simulink model "ModeInt"  (R2018b)
settings: Solver=FixedStepDiscrete  StartTime=0.0  StopTime=10.0  FixedStep=0.01  RelTol=1e-3
undefined symbols (not defined in the file or in its folder): c, CmprtMdHMIReqTp1, e, IfVeSMSeStNumConfig, MdReqTp1
(part 4 of 4)

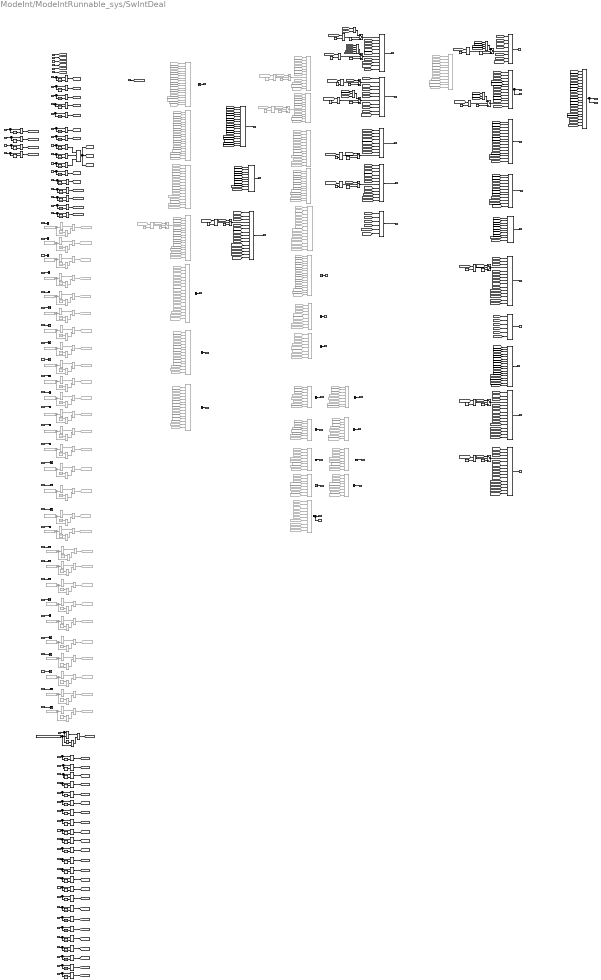
== system ModeInt/ModeIntRunnable_sys/SwIntDeal ==
  note: Note：
      | 1.修复Mode21/22/23/24自己硬线开关无法打断自己的问题。对应bug672425
  note: //local sw & memory sw & mode sw
  IsDrvStSwAct : Inport
  IsPasStSwAct : Inport  Port=2
  Is2LStSwAct : Inport  Port=3
  "Is2RStSwAct " : Inport  Port=4
  "Is3LStSwAct " : Inport  Port=5
  "Is3RStSwAct " : Inport  Port=6
  SwAcsExtLIntCnt : Inport  Port=7
  "SwAcsEntyLIntCnt " : Inport  Port=8
  "SwLfVipIntCnt " : Inport  Port=9
  SwRtVipIntCnt : Inport  Port=10
  SwLtLugIntCnt : Inport  Port=11
  SwRtLugIntCnt : Inport  Port=12
  SwAllLugIntCnt : Inport  Port=13
  SwLtRcvyIntCnt : Inport  Port=14
  SwRtRcvyIntCnt : Inport  Port=15
  AcsExtMdHMI2LRclReq : Inport  Port=16
  AcsExtMdHMI2RRclReq : Inport  Port=17
  VIPMdHMI2LRclReq : Inport  Port=18
  VIPMdHMI2RRclReq : Inport  Port=19
  RcvyMdHMI2LRclReq : Inport  Port=20
  RcvyMdHMI2RRclReq : Inport  Port=21
  LgrstOpenLtHMI2LRclReq : Inport  Port=22
  LgrstCloseLtHMI2LRclReq : Inport  Port=23
  LgrstOpenRtHMI2RRclReq : Inport  Port=24
  LgrstCloseRtHMI2RRclReq : Inport  Port=25
  passCmprtMdHMIReq : Inport  Port=26
  SRSAcsExtIntCnt : Inport  Port=27
  SRSAcsEntyIntCnt : Inport  Port=28
  SRSAllVipIntCnt : Inport  Port=29
  SRSAllLugIntCnt : Inport  Port=30
  SeStNumConfig : Inport  Port=31
  AcsEntryMdHMI2LRclReq : Inport  Port=32
  AcsEntryMdHMI2RRclReq : Inport  Port=33
  VipAllMdHMI2LRclReq : Inport  Port=34
  VipAllMdHMI2RRclReq : Inport  Port=35
  AllLugMdHMI2LRclReq : Inport  Port=36
  AllLugMdHMI2RRclReq : Inport  Port=37
  IntimacyLHMI2LRclReq : Inport  Port=38
  IntimacyRHMI2RRclReq : Inport  Port=39
  FamilyMdHMI2LRclReq : Inport  Port=40
  FamilyMdHMI2RRclReq : Inport  Port=41
  LtLugMdHMI2LRclReq : Inport  Port=42
  RtLugMdHMI2RRclReq : Inport  Port=43
  LtLyingMdHMI2LRclReq : Inport  Port=44
  RtLyingMdHMI2RRclReq : Inport  Port=45
  SRSLtFamilyIntCnt : Inport  Port=46
  SRSRtFamilyIntCnt : Inport  Port=47
  SRSIntimacyLtIntCnt : Inport  Port=48
  SRSIntimacyRtIntCnt : Inport  Port=49
  SRSLtLugIntCnt : Inport  Port=50
  SRSLtVipIntCnt : Inport  Port=51
  SRSLtLyingIntCnt : Inport  Port=52
  SRSRtLyingIntCnt : Inport  Port=53
  SRSLtRcvyIntCnt : Inport  Port=54
  SRSRtRcvyIntCnt : Inport  Port=55
  SRSRtLugIntCnt : Inport  Port=56
  SRSRtVipIntCnt : Inport  Port=57
  SRSLgrstOpenLtIntCnt : Inport  Port=58
  SRSLgrstCloseLtIntCnt : Inport  Port=59
  SRSLgrstOpenRtIntCnt : Inport  Port=60
  SRSLgrstCloseRtIntCnt : Inport  Port=61
  SwAcsExtRIntCnt : Inport  Port=62
  SwAcsEntyRIntCnt : Inport  Port=63
  SwAcsEntyBIntCnt_Val_read : Inport  Port=64
  SwAcsEntry4s2LIntCnt : Inport  Port=65
  SwAcsExit4s2LIntCnt : Inport  Port=66
  SwAcsEntry4s2RIntCnt : Inport  Port=67
  SwAcsExit4s2RIntCnt : Inport  Port=68
  AcsEntry4s2LHMI2LRclReq : Inport  Port=69
  AcsExit4s2LHMI2LRclReq : Inport  Port=70
  AcsEntry4s2RHMI2RRclReq : Inport  Port=71
  AcsExit4s2RHMI2RRclReq : Inport  Port=72
  SRSAcsEntry4s2LIntCnt : Inport  Port=73
  SRSAcsExit4s2LIntCnt : Inport  Port=74
  SRSAcsEntry4s2RIntCnt : Inport  Port=75
  SRSAcsExit4s2RIntCnt : Inport  Port=76
  SwPasReclinerEntryIntCnt : Inport  Port=77
  SwPasReclinerExitIntCnt : Inport  Port=78
  SwUnfold3LIntCnt : Inport  Port=79
  SwUnfold3RIntCnt : Inport  Port=80
  AND{,1,3..28} (28 alike) : Logic  Commented=on  AllPortsSameDT=off  OutDataTypeStr=boolean
  AND2 : Logic  AllPortsSameDT=off  OutDataTypeStr=boolean
  Constant{1,3..9,12..13,16..29,32..35} (28 alike) : Constant  Commented=on  Value=MdReqTp1.MdReqTp_Stop
  Constant10 : Constant  Commented=on  Value=IfVeSMSeStNumConfig.SeatNum7Config  OutDataTypeStr=Enum: IfVeSMSeStNumConfig
  Constant11 : Constant  Commented=on  Value=0  OutDataTypeStr=uint8
  Constant14 : Constant  Commented=on  Value=IfVeSMSeStNumConfig.SeatNum7Config  OutDataTypeStr=Enum: IfVeSMSeStNumConfig
  Constant15 : Constant  Commented=on  Value=0  OutDataTypeStr=uint8
  Constant2 : Constant  Value=CmprtMdHMIReqTp1.CmprtMdHMIReqTp_Stop  OutDataTypeStr=Enum:CmprtMdHMIReqTp1
  Constant30 : Constant  Commented=on  Value=IfVeSMSeStNumConfig.SeatNum7Config  OutDataTypeStr=Enum: IfVeSMSeStNumConfig
  Constant31 : Constant  Commented=on  Value=0  OutDataTypeStr=uint8
  Constant{36,38,40,42,44,46,48,50,52,54,56,58} (12 alike) : Constant  Value=IfVeSMSeStNumConfig.SeatNum7Config  OutDataTypeStr=Enum: IfVeSMSeStNumConfig
  Constant{37,39,41,43,45,47,49,51,53,55,57,59} (12 alike) : Constant  Value=0  OutDataTypeStr=uint8
  Equal{,1..8,14..18,27,32,59..69,79..88,97..104} (45 alike) : RelationalOperator  Operator=~=  OutDataTypeStr=boolean  RndMeth=Simplest
  Equal{10..11,19..20,23..24,28,33,35,37,39,41,43,45,47,49,51,53,55,57,71,73,75,77,90,92,94,96} (28 alike) : RelationalOperator  Commented=on  Operator=~=  OutDataTypeStr=boolean  RndMeth=Simplest
  Equal{13,105..116} (13 alike) : RelationalOperator  Operator===  OutDataTypeStr=boolean  RndMeth=Simplest
  Equal{9,12,21..22,25..26,29..31,34,36,38,40,42,44,46,48,50,52,54,56,58,70,72,74,76,78,89,91,93,95} (31 alike) : RelationalOperator  Commented=on  Operator===  OutDataTypeStr=boolean  RndMeth=Simplest
  From : From  Commented=on  GotoTag=IsDrvStSwAct
  From1 : From  Commented=on  GotoTag=IsPasStSwAct
  From{10,40,49,51,64,67,74,78,101,180,219,229,233,243} (14 alike) : From  Commented=on  GotoTag=SwAcsEntyRInt
  From{6,20,30,32,35,63,76,100,134,158,173,183,211..212} (14 alike) : From  Commented=on  GotoTag=SwAcsEntyLInt
  From102 : From  Commented=on  GotoTag=SRSAcsExtInt
  From103 : From  Commented=on  GotoTag=SRSAcsEntyInt
  From104 : From  Commented=on  GotoTag=SRSAllVipInt
  From105 : From  Commented=on  GotoTag=SRSAllLugInt
  From106 : From  Commented=on  GotoTag=AcsExtMdHMI2LStop
  From107 : From  Commented=on  GotoTag=VIPMdHMI2LStop
  From108 : From  Commented=on  GotoTag=RcvyMdHMI2LStop
  From109 : From  Commented=on  GotoTag=AcsExtMdHMI2RStop
  From{11,34,53,55,73,79,99,115,181,201,204,227,230,247} (14 alike) : From  Commented=on  GotoTag=SwAcsExtRInt
  From110 : From  Commented=on  GotoTag=VIPMdHMI2RStop
  From111 : From  Commented=on  GotoTag=RcvyMdHMI2RStop
  From{54,69,71,81,112..114,116,133,192,198,220,231,234} (14 alike) : From  Commented=on  GotoTag=SwAcsEntyBInt
  From117 : From  Commented=on  GotoTag=AcsEntryMdHMI2LStop
  From118 : From  Commented=on  GotoTag=AcsEntryMdHMI2RStop
  From119 : From  Commented=on  GotoTag=VipAllMdHMI2LStop
  From{12,23,36,61,137,164,178,186,195..196,207,238,271,279} (14 alike) : From  Commented=on  GotoTag=SwLtRcvyInt
  From120 : From  Commented=on  GotoTag=VipAllMdHMI2RStop
  From121 : From  Commented=on  GotoTag=AllLugMdHMI2LStop
  From122 : From  Commented=on  GotoTag=AllLugMdHMI2RStop
  From123 : From  Commented=on  GotoTag=IntimacyLHMI2LStop
  From{2,16,28,57,124,153,155,159,166,169,191,237,267,277} (14 alike) : From  Commented=on  GotoTag=Is2LStSwAct
  From125 : From  Commented=on  GotoTag=FamilyMdHMI2LStop
  From126 : From  Commented=on  GotoTag=FamilyMdHMI2RStop
  From127 : From  Commented=on  GotoTag=LtLugMdHMI2LStop
  From128 : From  Commented=on  GotoTag=RtLugMdHMI2RStop
  From129 : From  Commented=on  GotoTag=LtLyingMdHMI2LStop
  From{13,24,46,66,138,165,179,187,203,214,222,286,294..295} (14 alike) : From  Commented=on  GotoTag=SwRtRcvyInt
  From130 : From  Commented=on  GotoTag=RtLyingMdHMI2RStop
  From{5,26,52,131,156} (5 alike) : From  Commented=on  GotoTag=Is3RStSwAct
  From{3,17,38,62,132,152,154,167,170,199,218,270,284,292} (14 alike) : From  Commented=on  GotoTag=Is2RStSwAct
  From{7,21,31,39,44,60,135,160,163,174,184,190,194,206,236,266,278} (17 alike) : From  Commented=on  GotoTag=SwLfVipInt
  From{8,22,42,58..59,65,91,136,161,175,185,202,213,221,272,285,293} (17 alike) : From  Commented=on  GotoTag=SwRtVipInt
  From139 : From  Commented=on  GotoTag=SRSLtFamilyInt
  From14 : From  Commented=on  GotoTag=IsDrvStSwAct
  From140 : From  Commented=on  GotoTag=SRSRtFamilyInt
  From141 : From  Commented=on  GotoTag=SRSIntimacyLtInt
  From142 : From  Commented=on  GotoTag=SRSLtLugInt
  From{77,82,84,86,88,90,93..94,96,98,143,151,168,182,188,197,205,210,217,225,269,275,283,291} (24 alike) : From  Commented=on  GotoTag=passCmprtMdHMIStop
  From144 : From  Commented=on  GotoTag=SRSLtLyingInt
  From145 : From  Commented=on  GotoTag=SRSRtLyingInt
  From146 : From  Commented=on  GotoTag=SRSLtRcvyInt
  From147 : From  Commented=on  GotoTag=SRSRtRcvyInt
  From148 : From  Commented=on  GotoTag=SRSRtLugInt
  From149 : From  Commented=on  GotoTag=SRSLgrstOpenLtInt
  From15 : From  Commented=on  GotoTag=IsPasStSwAct
  From150 : From  Commented=on  GotoTag=LgrstOpenLtHMI2LStop
  From{18..19,29,45,48,68,75,92,157,172,177,193,200,226} (14 alike) : From  Commented=on  GotoTag=SwAcsExtLInt
  From162 : From  Commented=on  GotoTag=SeStNumConfig
  From{4,25,37,47,97,171} (6 alike) : From  Commented=on  GotoTag=Is3LStSwAct
  From{9,33,43,50,70,176,189,228,232,235} (10 alike) : From  Commented=on  GotoTag=SwLtLugInt
  From208 : From  Commented=on  GotoTag=SRSLgrstCloseLtInt
  From209 : From  Commented=on  GotoTag=LgrstCloseLtHMI2LStop
  From215 : From  Commented=on  GotoTag=SRSLgrstOpenRtInt
  From216 : From  Commented=on  GotoTag=LgrstOpenRtHMI2RStop
  From223 : From  Commented=on  GotoTag=SRSLgrstCloseRtInt
  From224 : From  Commented=on  GotoTag=LgrstCloseRtHMI2RStop
  From239 : From  Commented=on  GotoTag=AcsEntry4s2LHMI2LStop
  From{240,245,250,254,258,260,280,297,301} (9 alike) : From  Commented=on  GotoTag=SwAcsEntry4s2LInt
  From{241,246,251,255,259,261,276,296,300} (9 alike) : From  Commented=on  GotoTag=SwAcsExit4s2LInt
  From{242,248,252,256,262,264,287,299,302} (9 alike) : From  Commented=on  GotoTag=SwAcsEntry4s2RInt
  From{244,249,253,257,263,265,288,298,303} (9 alike) : From  Commented=on  GotoTag=SwAcsExit4s2RInt
  From268 : From  Commented=on  GotoTag=AcsExit4s2RHMI2RStop
  From27 : From  Commented=on  GotoTag=IntimacyRHMI2RStop
  From273 : From  Commented=on  GotoTag=SRSAcsExit4s2RInt
  From274 : From  Commented=on  GotoTag=SRSAcsEntry4s2LInt
  From281 : From  Commented=on  GotoTag=SRSAcsExit4s2LInt
  From282 : From  Commented=on  GotoTag=AcsExit4s2LHMI2LStop
  From289 : From  Commented=on  GotoTag=AcsEntry4s2RHMI2RStop
  From290 : From  Commented=on  GotoTag=SRSAcsEntry4s2RInt
  From41 : From  Commented=on  GotoTag=IsDrvStSwAct
  From56 : From  Commented=on  GotoTag=SwRtLugInt
  From72 : From  Commented=on  GotoTag=SwAllLugInt
  From80 : From  Commented=on  GotoTag=IsPasStSwAct
  From83 : From  Commented=on  GotoTag=SRSRtVipInt
  From85 : From  Commented=on  GotoTag=SRSLtVipInt
  From87 : From  Commented=on  GotoTag=SeStNumConfig
  From89 : From  Commented=on  GotoTag=SeStNumConfig
  From95 : From  Commented=on  GotoTag=SRSIntimacyRtInt
  Goto15 : Goto  Commented=on  GotoTag=AcsExtMdHMI2LStop
  Goto16 : Goto  Commented=on  GotoTag=AcsExtMdHMI2RStop
  Goto22 : Goto  Commented=on  GotoTag=VIPMdHMI2LStop
  Goto23 : Goto  Commented=on  GotoTag=VIPMdHMI2RStop
  Goto24 : Goto  Commented=on  GotoTag=RcvyMdHMI2LStop
  Goto25 : Goto  Commented=on  GotoTag=RcvyMdHMI2RStop
  Goto26 : Goto  Commented=on  GotoTag=LgrstOpenLtHMI2LStop
  Goto27 : Goto  Commented=on  GotoTag=LgrstCloseLtHMI2LStop
  Goto29 : Goto  Commented=on  GotoTag=AcsEntryMdHMI2LStop
  Goto30 : Goto  Commented=on  GotoTag=AcsEntryMdHMI2RStop
  Goto31 : Goto  Commented=on  GotoTag=VipAllMdHMI2LStop
  Goto32 : Goto  Commented=on  GotoTag=VipAllMdHMI2RStop
  Goto33 : Goto  Commented=on  GotoTag=AllLugMdHMI2LStop
  Goto34 : Goto  Commented=on  GotoTag=AllLugMdHMI2RStop
  Goto35 : Goto  Commented=on  GotoTag=IntimacyLHMI2LStop
  Goto36 : Goto  Commented=on  GotoTag=IntimacyRHMI2RStop
  Goto37 : Goto  Commented=on  GotoTag=FamilyMdHMI2LStop
  Goto38 : Goto  Commented=on  GotoTag=FamilyMdHMI2RStop
  Goto39 : Goto  Commented=on  GotoTag=LtLugMdHMI2LStop
  Goto40 : Goto  Commented=on  GotoTag=RtLugMdHMI2RStop
  Goto41 : Goto  Commented=on  GotoTag=LtLyingMdHMI2LStop
  Goto42 : Goto  Commented=on  GotoTag=RtLyingMdHMI2RStop
  Goto54 : Goto  Commented=on  GotoTag=LgrstOpenRtHMI2RStop
  Goto55 : Goto  Commented=on  GotoTag=LgrstCloseRtHMI2RStop
  Goto68 : Goto  Commented=on  GotoTag=AcsEntry4s2LHMI2LStop
  Goto69 : Goto  Commented=on  GotoTag=AcsExit4s2LHMI2LStop
  Goto70 : Goto  Commented=on  GotoTag=AcsEntry4s2RHMI2RStop
  Goto71 : Goto  Commented=on  GotoTag=AcsExit4s2RHMI2RStop
  Ground{,1..15} (16 alike) : Ground
  OR : Logic  Commented=on  Operator=OR  Inputs=20  AllPortsSameDT=off  OutDataTypeStr=boolean
  OR1 : Logic  Commented=on  Operator=OR  Inputs=18  AllPortsSameDT=off  OutDataTypeStr=boolean
  OR10 : Logic  Commented=on  Operator=OR  Inputs=15  AllPortsSameDT=off  OutDataTypeStr=boolean
  OR{11,16..24} (10 alike) : Logic  Commented=on  Operator=OR  Inputs=8  AllPortsSameDT=off  OutDataTypeStr=boolean
  OR12 : Logic  Operator=OR  Inputs=3  AllPortsSameDT=off  OutDataTypeStr=boolean
  OR13 : Logic  Commented=on  Operator=OR  Inputs=17  AllPortsSameDT=off  OutDataTypeStr=boolean
  OR14 : Logic  Commented=on  Operator=OR  Inputs=17  AllPortsSameDT=off  OutDataTypeStr=boolean
  OR15 : Logic  Commented=on  Operator=OR  Inputs=15  AllPortsSameDT=off  OutDataTypeStr=boolean
  OR2 : Logic  Commented=on  Operator=OR  Inputs=16  AllPortsSameDT=off  OutDataTypeStr=boolean
  OR25 : Logic  Commented=on  Operator=OR  Inputs=10  AllPortsSameDT=off  OutDataTypeStr=boolean
  OR26 : Logic  Operator=OR  Inputs=17  AllPortsSameDT=off  OutDataTypeStr=boolean
  OR27 : Logic  Operator=OR  Inputs=10  AllPortsSameDT=off  OutDataTypeStr=boolean
  OR{28,40,43,45..46} (5 alike) : Logic  Operator=OR  Inputs=15  AllPortsSameDT=off  OutDataTypeStr=boolean
  OR29 : Logic  Operator=OR  AllPortsSameDT=off  OutDataTypeStr=boolean
  OR3 : Logic  Commented=on  Operator=OR  Inputs=17  AllPortsSameDT=off  OutDataTypeStr=boolean
  OR30 : Logic  Operator=OR  Inputs=5  AllPortsSameDT=off  OutDataTypeStr=boolean
  OR31 : Logic  Operator=OR  Inputs=11  AllPortsSameDT=off  OutDataTypeStr=boolean
  OR32 : Logic  Operator=OR  Inputs=17  AllPortsSameDT=off  OutDataTypeStr=boolean
  OR33 : Logic  Operator=OR  Inputs=11  AllPortsSameDT=off  OutDataTypeStr=boolean
  OR34 : Logic  Operator=OR  Inputs=9  AllPortsSameDT=off  OutDataTypeStr=boolean
  OR35 : Logic  Operator=OR  Inputs=12  AllPortsSameDT=off  OutDataTypeStr=boolean
  OR36 : Logic  Operator=OR  Inputs=6  AllPortsSameDT=off  OutDataTypeStr=boolean
  OR37 : Logic  Operator=OR  Inputs=8  AllPortsSameDT=off  OutDataTypeStr=boolean
  OR38 : Logic  Operator=OR  Inputs=4  AllPortsSameDT=off  OutDataTypeStr=boolean
  OR39 : Logic  Operator=OR  Inputs=13  AllPortsSameDT=off  OutDataTypeStr=boolean
  OR4 : Logic  Commented=on  Operator=OR  Inputs=12  AllPortsSameDT=off  OutDataTypeStr=boolean
  OR41 : Logic  Operator=OR  Inputs=12  AllPortsSameDT=off  OutDataTypeStr=boolean
  OR42 : Logic  Operator=OR  Inputs=10  AllPortsSameDT=off  OutDataTypeStr=boolean
  OR44 : Logic  Operator=OR  Inputs=6  AllPortsSameDT=off  OutDataTypeStr=boolean
  OR47 : Logic  Operator=OR  Inputs=3  AllPortsSameDT=off  OutDataTypeStr=boolean
  OR48 : Logic  Operator=OR  Inputs=3  AllPortsSameDT=off  OutDataTypeStr=boolean
  OR49 : Logic  Operator=OR  Inputs=20  AllPortsSameDT=off  OutDataTypeStr=boolean
  OR5 : Logic  Commented=on  Operator=OR  Inputs=12  AllPortsSameDT=off  OutDataTypeStr=boolean
  OR6 : Logic  Commented=on  Operator=OR  Inputs=13  AllPortsSameDT=off  OutDataTypeStr=boolean
  OR7 : Logic  Commented=on  Operator=OR  Inputs=13  AllPortsSameDT=off  OutDataTypeStr=boolean
  OR8 : Logic  Commented=on  Operator=OR  Inputs=14  AllPortsSameDT=off  OutDataTypeStr=boolean
  OR9 : Logic  Commented=on  Operator=OR  Inputs=12  AllPortsSameDT=off  OutDataTypeStr=boolean
  Switch : Switch  Commented=on  Criteria=u2 > Threshold
  Switch1 : Switch  Commented=on  Criteria=u2 > Threshold
  Switch{3..13,15} (12 alike) : Switch  Criteria=u2 > Threshold
  Switch2 : Switch  Commented=on  Criteria=u2 > Threshold
  Terminator{,1..27} (28 alike) : Terminator
  Unit Delay{,1..8,12..15,34..44,49..60,65..72} (44 alike) : UnitDelay  SampleTime=-1
  Unit Delay{9..10,16..33,45..48,61..64} (28 alike) : UnitDelay  Commented=on  InitialCondition=e  SampleTime=-1
  Unit Delay11 : UnitDelay  InitialCondition=c  SampleTime=-1
  SwIntAcsEnty : Outport
  SwIntAcsExt : Outport  Port=2
  SwIntLfVip : Outport  Port=3
  SwIntRtVip : Outport  Port=4
  SwIntLfLug : Outport  Port=5
  SwIntRtLug : Outport  Port=6
  SwIntLfRcvy : Outport  Port=7
  SwIntRtRcvy : Outport  Port=8
  SwIntAllVip : Outport  Port=9
  SwIntAllLug : Outport  Port=10
  SwIntLtFamily : Outport  Port=11
  SwIntRtFamily : Outport  Port=12
  SwIntIntimacyLt : Outport  Port=13
  SwIntLtLying : Outport  Port=14
  SwIntRtLying : Outport  Port=15
  SwIntIntimacyRt : Outport  Port=16
  SwIntLgrstOpenLt : Outport  Port=17
  SwIntLgrstCloseLt : Outport  Port=18
  SwIntLgrstOpenRt : Outport  Port=19
  SwIntLgrstCloseRt : Outport  Port=20
  SwIntAcsEntry4s2L : Outport  Port=21
  SwIntAcsExit4s2L : Outport  Port=22
  SwIntAcsEntry4s2R : Outport  Port=23
  SwIntAcsExit4s2R : Outport  Port=24
  SwIntAcsEntryAll4sBwd : Outport  Port=25
  SwIntAcsEntryAll4sFwd : Outport  Port=26
  SwIntPasReclinerEntry : Outport  Port=27
  SwIntPasReclinerExit : Outport  Port=28
  SwIntUnfold3L : Outport  Port=29
  SwIntUnfold3R : Outport  Port=30
  SwIntLfVipOut : Outport  Port=31
  SwIntRtVipOut : Outport  Port=32
  SwIntAllVipOut : Outport  Port=33
  SwIntBig4Seat : Outport  Port=34
  SwIntExVIPR : Outport  Port=35
  SwIntExVIPROut : Outport  Port=36
  SwIntWholeVehMem1 : Outport  Port=37
  SwIntWholeVehMem2 : Outport  Port=38
  wires:
  IsDrvStSwAct/1 -> [IsDrvStSwAct]
  IsPasStSwAct/1 -> [IsPasStSwAct]
  Is2LStSwAct/1 -> [Is2LStSwAct]
  "Is2RStSwAct "/1 -> [Is2RStSwAct]
  "Is3LStSwAct "/1 -> [Is3LStSwAct]
  "Is3RStSwAct "/1 -> [Is3RStSwAct]
  From/1 -> OR/1
  From1/1 -> OR/2
  From2/1 -> OR/3
  From3/1 -> OR/4
  From4/1 -> OR/5
  From5/1 -> OR/6
  From14/1 -> OR1/1
  From15/1 -> OR1/2
  From16/1 -> OR1/3
  From17/1 -> OR1/4
  From52/1 -> OR5/1
  From57/1 -> OR6/1
  From62/1 -> OR7/1
  Equal2/1 -> [SwLfVipInt]
  "SwLfVipIntCnt "/1 -> Equal2/1, Unit Delay2/1
  Unit Delay2/1 -> Equal2/2
  SwRtVipIntCnt/1 -> Unit Delay3/1, Equal3/1
  Unit Delay3/1 -> Equal3/2
  Equal3/1 -> [SwRtVipInt]
  SwLtLugIntCnt/1 -> Equal4/1, Unit Delay4/1
  Unit Delay4/1 -> Equal4/2
  SwRtLugIntCnt/1 -> Unit Delay5/1, Equal5/1
  Unit Delay5/1 -> Equal5/2
  Unit Delay6/1 -> Equal6/2
  SwAllLugIntCnt/1 -> Unit Delay6/1, Equal6/1
  Equal7/1 -> [SwLtRcvyInt]
  SwLtRcvyIntCnt/1 -> Unit Delay7/1, Equal7/1
  Unit Delay7/1 -> Equal7/2
  Equal8/1 -> [SwRtRcvyInt]
  SwRtRcvyIntCnt/1 -> Unit Delay8/1, Equal8/1
  Unit Delay8/1 -> Equal8/2
  Constant8/1 -> Equal10/2, Equal9/2
  Unit Delay9/1 -> Equal10/1
  Equal9/1 -> AND/1
  Equal10/1 -> AND/2
  AND/1 -> Goto15/1
  Constant1/1 -> Equal11/2, Equal12/2
  AND1/1 -> Goto16/1
  Unit Delay10/1 -> Equal11/1
  Equal11/1 -> AND1/2
  Equal12/1 -> AND1/1
  passCmprtMdHMIReq/1 -> Unit Delay11/1, Equal13/1
  Constant2/1 -> Equal14/2, Equal13/2
  Unit Delay11/1 -> Equal14/1
  Equal13/1 -> AND2/1
  Equal14/1 -> AND2/2
  AND2/1 -> [passCmprtMdHMIStop]
  Unit Delay15/1 -> Equal18/2
  SRSAllVipIntCnt/1 -> Unit Delay14/1, Equal17/1
  SRSAllLugIntCnt/1 -> Unit Delay15/1, Equal18/1
  SRSAcsEntyIntCnt/1 -> Unit Delay13/1, Equal16/1
  SRSAcsExtIntCnt/1 -> Unit Delay12/1, Equal15/1
  Unit Delay14/1 -> Equal17/2
  Unit Delay13/1 -> Equal16/2
  Equal18/1 -> [SRSAllLugInt]
  Equal15/1 -> [SRSAcsExtInt]
  Unit Delay12/1 -> Equal15/2
  Equal17/1 -> [SRSAllVipInt]
  Equal16/1 -> [SRSAcsEntyInt]
  Equal22/1 -> AND3/1
  AND4/1 -> Goto23/1
  AND3/1 -> Goto22/1
  Constant4/1 -> Equal19/2, Equal22/2
  Equal19/1 -> AND3/2
  Unit Delay16/1 -> Equal20/1
  Equal21/1 -> AND4/1
  Equal20/1 -> AND4/2
  Unit Delay17/1 -> Equal19/1
  Constant3/1 -> Equal20/2, Equal21/2
  Equal25/1 -> AND6/1
  Constant5/1 -> Equal24/2, Equal25/2
  Unit Delay19/1 -> Equal23/1
  Constant6/1 -> Equal23/2, Equal26/2
  AND5/1 -> Goto24/1
  Equal23/1 -> AND5/2
  Unit Delay18/1 -> Equal24/1
  Equal26/1 -> AND5/1
  AND6/1 -> Goto25/1
  Equal24/1 -> AND6/2
  AND7/1 -> Goto29/1
  Equal30/1 -> AND7/1
  Equal28/1 -> AND7/2
  Constant7/1 -> Equal28/2, Equal30/2
  Unit Delay20/1 -> Equal28/1
  Unit Delay21/1 -> Equal33/1
  Constant9/1 -> Equal33/2, Equal34/2
  Equal34/1 -> AND8/1
  Equal33/1 -> AND8/2
  AND8/1 -> Goto30/1
  AND9/1 -> Goto31/1
  Constant12/1 -> Equal35/2, Equal36/2
  Equal36/1 -> AND9/1
  Unit Delay22/1 -> Equal35/1
  Equal35/1 -> AND9/2
  Constant13/1 -> Equal37/2, Equal38/2
  AND10/1 -> Goto32/1
  Unit Delay23/1 -> Equal37/1
  Equal38/1 -> AND10/1
  Equal37/1 -> AND10/2
  AND11/1 -> Goto33/1
  Equal39/1 -> AND11/2
  Unit Delay24/1 -> Equal39/1
  Equal40/1 -> AND11/1
  Constant20/1 -> Equal39/2, Equal40/2
  Constant21/1 -> Equal41/2, Equal42/2
  Equal42/1 -> AND12/1
  Equal41/1 -> AND12/2
  Unit Delay25/1 -> Equal41/1
  AND12/1 -> Goto34/1
  Equal44/1 -> AND13/1
  Unit Delay26/1 -> Equal43/1
  Constant22/1 -> Equal43/2, Equal44/2
  AND13/1 -> Goto35/1
  Equal43/1 -> AND13/2
  Equal45/1 -> AND14/2
  Constant23/1 -> Equal45/2, Equal46/2
  Unit Delay27/1 -> Equal45/1
  AND14/1 -> Goto36/1
  Equal46/1 -> AND14/1
  Equal48/1 -> AND15/1
  AND15/1 -> Goto37/1
  Unit Delay28/1 -> Equal47/1
  Constant24/1 -> Equal47/2, Equal48/2
  Equal47/1 -> AND15/2
  Equal50/1 -> AND16/1
  AND16/1 -> Goto38/1
  Equal49/1 -> AND16/2
  Unit Delay29/1 -> Equal49/1
  Constant25/1 -> Equal49/2, Equal50/2
  Constant26/1 -> Equal51/2, Equal52/2
  Unit Delay30/1 -> Equal51/1
  AND17/1 -> Goto39/1
  Equal51/1 -> AND17/2
  Equal52/1 -> AND17/1
  AND18/1 -> Goto40/1
  Unit Delay31/1 -> Equal53/1
  Equal54/1 -> AND18/1
  Equal53/1 -> AND18/2
  Constant27/1 -> Equal53/2, Equal54/2
  Constant28/1 -> Equal55/2, Equal56/2
  Equal55/1 -> AND19/2
  Unit Delay32/1 -> Equal55/1
  Equal56/1 -> AND19/1
  AND19/1 -> Goto41/1
  Constant29/1 -> Equal57/2, Equal58/2
  Equal57/1 -> AND20/2
  Unit Delay33/1 -> Equal57/1
  Equal58/1 -> AND20/1
  AND20/1 -> Goto42/1
  Equal59/1 -> [SRSLtFamilyInt]
  SRSLtFamilyIntCnt/1 -> Unit Delay34/1, Equal59/1
  Unit Delay34/1 -> Equal59/2
  Unit Delay35/1 -> Equal60/2
  Equal60/1 -> [SRSRtFamilyInt]
  SRSRtFamilyIntCnt/1 -> Unit Delay35/1, Equal60/1
  Unit Delay36/1 -> Equal61/2
  SRSIntimacyLtIntCnt/1 -> Unit Delay36/1, Equal61/1
  Equal61/1 -> [SRSIntimacyLtInt]
  Equal62/1 -> [SRSLtLugInt]
  SRSLtLugIntCnt/1 -> Unit Delay37/1, Equal62/1
  Unit Delay37/1 -> Equal62/2
  Unit Delay38/1 -> Equal63/2
  SRSLtVipIntCnt/1 -> Unit Delay38/1, Equal63/1
  Equal63/1 -> [SRSLtVipInt]
  Equal64/1 -> [SRSLtLyingInt]
  SRSLtLyingIntCnt/1 -> Unit Delay39/1, Equal64/1
  Unit Delay39/1 -> Equal64/2
  Unit Delay40/1 -> Equal65/2
  Equal65/1 -> [SRSRtLyingInt]
  SRSRtLyingIntCnt/1 -> Unit Delay40/1, Equal65/1
  SRSLtRcvyIntCnt/1 -> Unit Delay41/1, Equal66/1
  Equal66/1 -> [SRSLtRcvyInt]
  Unit Delay41/1 -> Equal66/2
  SRSRtRcvyIntCnt/1 -> Unit Delay42/1, Equal67/1
  Unit Delay42/1 -> Equal67/2
  Equal67/1 -> [SRSRtRcvyInt]
  Unit Delay43/1 -> Equal68/2
  Equal68/1 -> [SRSRtLugInt]
  SRSRtLugIntCnt/1 -> Unit Delay43/1, Equal68/1
  Unit Delay44/1 -> Equal69/2
  Equal69/1 -> [SRSRtVipInt]
  SRSRtVipIntCnt/1 -> Unit Delay44/1, Equal69/1
  From153/1 -> OR13/1
  From154/1 -> OR13/2
  From171/1 -> OR14/3
  From170/1 -> OR14/2
  From169/1 -> OR14/1
  From159/1 -> OR15/1
  From167/1 -> OR15/2
  From191/1 -> OR16/1
  From199/1 -> OR17/1
  "SwAcsEntyLIntCnt "/1 -> Unit Delay1/1, Equal1/1
  Unit Delay1/1 -> Equal1/2
  Equal1/1 -> [SwAcsEntyLInt]
  Unit Delay/1 -> Equal/2
  SwAcsExtLIntCnt/1 -> Unit Delay/1, Equal/1
  Equal/1 -> [SwAcsExtLInt]
  From156/1 -> OR13/4
  From97/1 -> OR13/3
  From131/1 -> OR14/4
  Equal72/1 -> AND21/1
  Unit Delay45/1 -> Equal71/1
  Equal71/1 -> AND21/2
  Constant32/1 -> Equal71/2, Equal72/2
  AND21/1 -> Goto26/1
  Constant33/1 -> Equal73/2, Equal74/2
  Equal73/1 -> AND22/2
  Equal74/1 -> AND22/1
  Unit Delay46/1 -> Equal73/1
  AND22/1 -> Goto27/1
  Constant34/1 -> Equal75/2, Equal76/2
  Equal75/1 -> AND23/2
  Equal76/1 -> AND23/1
  Unit Delay47/1 -> Equal75/1
  AND23/1 -> Goto54/1
  Unit Delay48/1 -> Equal77/1
  AND24/1 -> Goto55/1
  Equal78/1 -> AND24/1
  Equal77/1 -> AND24/2
  Constant35/1 -> Equal77/2, Equal78/2
  Unit Delay49/1 -> Equal79/2
  SRSIntimacyRtIntCnt/1 -> Unit Delay49/1, Equal79/1
  Equal79/1 -> [SRSIntimacyRtInt]
  Equal80/1 -> [SRSLgrstOpenLtInt]
  SRSLgrstOpenLtIntCnt/1 -> Unit Delay50/1, Equal80/1
  Unit Delay50/1 -> Equal80/2
  Unit Delay51/1 -> Equal81/2
  Equal81/1 -> [SRSLgrstCloseLtInt]
  SRSLgrstCloseLtIntCnt/1 -> Unit Delay51/1, Equal81/1
  SRSLgrstOpenRtIntCnt/1 -> Unit Delay52/1, Equal82/1
  Equal82/1 -> [SRSLgrstOpenRtInt]
  Unit Delay52/1 -> Equal82/2
  Equal83/1 -> [SRSLgrstCloseRtInt]
  SRSLgrstCloseRtIntCnt/1 -> Unit Delay53/1, Equal83/1
  Unit Delay53/1 -> Equal83/2
  From132/1 -> OR10/2
  From124/1 -> OR10/1
  From166/1 -> OR11/1
  From155/1 -> OR18/1
  From152/1 -> OR19/1
  From218/1 -> OR20/1
  SeStNumConfig/1 -> [SeStNumConfig]
  From89/1 -> Equal70/1
  Constant30/1 -> Equal70/2
  Constant31/1 -> Switch1/3
  Equal70/1 -> Switch1/2
  From37/1 -> Switch1/1
  From25/1 -> OR2/3
  From28/1 -> OR2/2
  From41/1 -> OR2/1
  Unit Delay54/1 -> Equal27/2
  SwAcsExtRIntCnt/1 -> Unit Delay54/1, Equal27/1
  Equal27/1 -> [SwAcsExtRInt]
  Unit Delay55/1 -> Equal84/2
  SwAcsEntyRIntCnt/1 -> Unit Delay55/1, Equal84/1
  Equal84/1 -> [SwAcsEntyRInt]
  From19/1 -> OR1/5
  From34/1 -> OR1/6
  From20/1 -> OR1/7
  From51/1 -> OR1/8
  From21/1 -> OR1/9
  From22/1 -> OR1/10
  From23/1 -> OR1/11
  From24/1 -> OR1/12
  From26/1 -> OR3/3
  From38/1 -> OR3/2
  From80/1 -> OR3/1
  Switch1/1 -> OR3/4
  Unit Delay56/1 -> Equal85/2
  SwAcsEntyBIntCnt_Val_read/1 -> Unit Delay56/1, Equal85/1
  Equal85/1 -> [SwAcsEntyBInt]
  From81/1 -> OR/11
  From74/1 -> OR/10
  From6/1 -> OR/9
  From73/1 -> OR/8
  From18/1 -> OR/7
  From7/1 -> OR/12
  From8/1 -> OR/13
  From9/1 -> OR/14
  From30/1 -> OR2/4
  From107/1 -> OR2/12
  From90/1 -> OR2/13
  From85/1 -> OR2/14
  From110/1 -> OR3/14
  From88/1 -> OR3/15
  From158/1 -> OR13/5
  From183/1 -> OR15/3
  From134/1 -> OR10/3
  From212/1 -> OR8/1
  From243/1 -> OR8/2
  From234/1 -> OR8/3
  From68/1 -> OR9/1
  From79/1 -> OR9/2
  From72/1 -> OR9/6
  From69/1 -> OR9/5
  From49/1 -> OR9/4
  From32/1 -> OR9/3
  From70/1 -> OR1/13
  From84/1 -> OR1/17
  From102/1 -> OR1/14
  From106/1 -> OR1/15
  From109/1 -> OR1/16
  From71/1 -> OR1/18
  From13/1 -> OR/16
  From12/1 -> OR/15
  From103/1 -> OR/17
  From117/1 -> OR/18
  From118/1 -> OR/19
  From86/1 -> OR/20
  From10/1 -> OR2/5
  From112/1 -> OR2/6
  From29/1 -> OR2/7
  From11/1 -> OR2/8
  From31/1 -> OR2/9
  From33/1 -> OR2/10
  From36/1 -> OR2/11
  From75/1 -> OR3/5
  From115/1 -> OR3/6
  From35/1 -> OR3/7
  From40/1 -> OR3/8
  From114/1 -> OR3/9
  From42/1 -> OR3/10
  From46/1 -> OR3/11
  From43/1 -> OR3/12
  From83/1 -> OR3/13
  From226/1 -> OR8/4
  From247/1 -> OR8/5
  From235/1 -> OR8/6
  From104/1 -> OR8/7
  From119/1 -> OR8/8
  From120/1 -> OR8/9
  From82/1 -> OR8/10
  From45/1 -> OR5/2
  From53/1 -> OR5/3
  From76/1 -> OR5/4
  From78/1 -> OR5/5
  From54/1 -> OR5/6
  From92/1 -> OR6/2
  From99/1 -> OR6/3
  From100/1 -> OR6/4
  From101/1 -> OR6/5
  From113/1 -> OR6/6
  From60/1 -> OR6/7
  From61/1 -> OR6/8
  From200/1 -> OR7/2
  From201/1 -> OR7/3
  From211/1 -> OR7/4
  From219/1 -> OR7/5
  From220/1 -> OR7/6
  From65/1 -> OR7/7
  From66/1 -> OR7/8
  From64/1 -> OR13/6
  From116/1 -> OR13/7
  From227/1 -> OR13/9
  From157/1 -> OR13/8
  From160/1 -> OR13/10
  From161/1 -> OR13/11
  From164/1 -> OR13/12
  From165/1 -> OR13/13
  From228/1 -> OR13/14
  From139/1 -> OR13/15
  From125/1 -> OR13/16
  From168/1 -> OR13/17
  From173/1 -> OR14/5
  From229/1 -> OR14/6
  From231/1 -> OR14/7
  From172/1 -> OR14/8
  From230/1 -> OR14/9
  From174/1 -> OR14/10
  From175/1 -> OR14/11
  From178/1 -> OR14/12
  From179/1 -> OR14/13
  From176/1 -> OR14/14
  From140/1 -> OR14/15
  From126/1 -> OR14/16
  From182/1 -> OR14/17
  From194/1 -> OR16/2
  From195/1 -> OR16/3
  From144/1 -> OR16/4
  From129/1 -> OR16/5
  From197/1 -> OR16/6
  From202/1 -> OR17/2
  From203/1 -> OR17/3
  From145/1 -> OR17/4
  From130/1 -> OR17/5
  From205/1 -> OR17/6
  From190/1 -> OR11/2
  From196/1 -> OR11/3
  From149/1 -> OR11/4
  From150/1 -> OR11/5
  From151/1 -> OR11/6
  From206/1 -> OR18/2
  From207/1 -> OR18/3
  From208/1 -> OR18/4
  From209/1 -> OR18/5
  From210/1 -> OR18/6
  From213/1 -> OR19/2
  From214/1 -> OR19/3
  From215/1 -> OR19/4
  From216/1 -> OR19/5
  From217/1 -> OR19/6
  From221/1 -> OR20/2
  From222/1 -> OR20/3
  From223/1 -> OR20/4
  From224/1 -> OR20/5
  From225/1 -> OR20/6
  Equal5/1 -> OR12/2
  Equal4/1 -> OR12/1
  Equal6/1 -> OR12/3
  OR12/1 -> [SwAllLugInt], [SwRtLugInt], [SwLtLugInt]
  From146/1 -> OR6/9
  From108/1 -> OR6/10
  From96/1 -> OR6/11
  From147/1 -> OR7/9
  From111/1 -> OR7/10
  From98/1 -> OR7/11
  From47/1 -> OR4/1
  From48/1 -> OR4/2
  From55/1 -> OR4/3
  From63/1 -> OR4/4
  From67/1 -> OR4/5
  From198/1 -> OR4/6
  From39/1 -> OR4/7
  Constant10/1 -> Equal29/2
  From87/1 -> Equal29/1
  From59/1 -> Switch/1
  Equal29/1 -> Switch/2
  Constant11/1 -> Switch/3
  Switch/1 -> OR4/8
  From50/1 -> OR4/9
  Constant15/1 -> Switch2/3
  Equal31/1 -> Switch2/2
  From163/1 -> Switch2/1
  From162/1 -> Equal31/1
  Constant14/1 -> Equal31/2
  Switch2/1 -> OR5/7
  From91/1 -> OR5/8
  From56/1 -> OR5/9
  From142/1 -> OR4/10
  From127/1 -> OR4/11
  From93/1 -> OR4/12
  From148/1 -> OR5/10
  From128/1 -> OR5/11
  From94/1 -> OR5/12
  From58/1 -> OR9/8
  From44/1 -> OR9/7
  From105/1 -> OR9/9
  From121/1 -> OR9/10
  From122/1 -> OR9/11
  From77/1 -> OR9/12
  From233/1 -> OR15/4
  From133/1 -> OR15/5
  From177/1 -> OR15/6
  From181/1 -> OR15/7
  From186/1 -> OR15/8
  From187/1 -> OR15/9
  From184/1 -> OR15/10
  From185/1 -> OR15/11
  From189/1 -> OR15/12
  From141/1 -> OR15/13
  From123/1 -> OR15/14
  From188/1 -> OR15/15
  From180/1 -> OR10/4
  From192/1 -> OR10/5
  From193/1 -> OR10/6
  From204/1 -> OR10/7
  From135/1 -> OR10/8
  From136/1 -> OR10/9
  From137/1 -> OR10/10
  From138/1 -> OR10/11
  From232/1 -> OR10/12
  From95/1 -> OR10/13
  From27/1 -> OR10/14
  From143/1 -> OR10/15
  SwAcsEntry4s2LIntCnt/1 -> Unit Delay57/1, Equal32/1
  Unit Delay57/1 -> Equal32/2
  Equal32/1 -> [SwAcsEntry4s2LInt]
  SwAcsExit4s2LIntCnt/1 -> Unit Delay58/1, Equal86/1
  Unit Delay58/1 -> Equal86/2
  Equal86/1 -> [SwAcsExit4s2LInt]
  SwAcsEntry4s2RIntCnt/1 -> Unit Delay59/1, Equal87/1
  Unit Delay59/1 -> Equal87/2
  Equal87/1 -> [SwAcsEntry4s2RInt]
  SwAcsExit4s2RIntCnt/1 -> Unit Delay60/1, Equal88/1
  Unit Delay60/1 -> Equal88/2
  Equal88/1 -> [SwAcsExit4s2RInt]
  Constant16/1 -> Equal90/2, Equal89/2
  Unit Delay61/1 -> Equal90/1
  Equal89/1 -> AND25/1
  Equal90/1 -> AND25/2
  AND25/1 -> Goto68/1
  Constant17/1 -> Equal92/2, Equal91/2
  Unit Delay62/1 -> Equal92/1
  Equal91/1 -> AND26/1
  Equal92/1 -> AND26/2
  AND26/1 -> Goto69/1
  Constant18/1 -> Equal94/2, Equal93/2
  Unit Delay63/1 -> Equal94/1
  Equal93/1 -> AND27/1
  Equal94/1 -> AND27/2
  AND27/1 -> Goto70/1
  Constant19/1 -> Equal96/2, Equal95/2
  Unit Delay64/1 -> Equal96/1
  Equal95/1 -> AND28/1
  Equal96/1 -> AND28/2
  AND28/1 -> Goto71/1
  SRSAcsEntry4s2LIntCnt/1 -> Unit Delay65/1, Equal97/1
  Unit Delay65/1 -> Equal97/2
  Equal97/1 -> [SRSAcsEntry4s2LInt]
  SRSAcsExit4s2LIntCnt/1 -> Unit Delay66/1, Equal98/1
  Unit Delay66/1 -> Equal98/2
  Equal98/1 -> [SRSAcsExit4s2LInt]
  SRSAcsEntry4s2RIntCnt/1 -> Unit Delay67/1, Equal99/1
  Unit Delay67/1 -> Equal99/2
  Equal99/1 -> [SRSAcsEntry4s2RInt]
  SRSAcsExit4s2RIntCnt/1 -> Unit Delay68/1, Equal100/1
  Unit Delay68/1 -> Equal100/2
  Equal100/1 -> [SRSAcsExit4s2RInt]
  From240/1 -> OR2/15
  From241/1 -> OR2/16
  From242/1 -> OR3/16
  From244/1 -> OR3/17
  From245/1 -> OR6/12
  From246/1 -> OR6/13
  From248/1 -> OR7/12
  From249/1 -> OR7/13
  From301/1 -> OR8/11
  From300/1 -> OR8/12
  From252/1 -> OR8/13
  From253/1 -> OR8/14
  From254/1 -> OR16/7
  From255/1 -> OR16/8
  From256/1 -> OR17/7
  From257/1 -> OR17/8
  From258/1 -> OR11/7
  From259/1 -> OR11/8
  From260/1 -> OR18/7
  From261/1 -> OR18/8
  From262/1 -> OR19/7
  From263/1 -> OR19/8
  From264/1 -> OR20/7
  From265/1 -> OR20/8
  From237/1 -> OR21/1
  From236/1 -> OR21/2
  From238/1 -> OR21/3
  From276/1 -> OR21/4
  From277/1 -> OR22/1
  From278/1 -> OR22/2
  From279/1 -> OR22/3
  From280/1 -> OR22/4
  From284/1 -> OR23/1
  From285/1 -> OR23/2
  From286/1 -> OR23/3
  From288/1 -> OR23/4
  From292/1 -> OR24/1
  From293/1 -> OR24/2
  From294/1 -> OR24/3
  From287/1 -> OR24/4
  From299/1 -> OR25/10
  From298/1 -> OR25/9
  From297/1 -> OR25/8
  From296/1 -> OR25/7
  From295/1 -> OR25/6
  From272/1 -> OR25/5
  From271/1 -> OR25/4
  From266/1 -> OR25/3
  From270/1 -> OR25/2
  From267/1 -> OR25/1
  From275/1 -> OR21/8
  From239/1 -> OR21/7
  From274/1 -> OR21/6
  From250/1 -> OR21/5
  From283/1 -> OR22/8
  From282/1 -> OR22/7
  From281/1 -> OR22/6
  From251/1 -> OR22/5
  From291/1 -> OR23/8
  From290/1 -> OR23/7
  From289/1 -> OR23/6
  From302/1 -> OR23/5
  From269/1 -> OR24/8
  From273/1 -> OR24/7
  From268/1 -> OR24/6
  From303/1 -> OR24/5
  Unit Delay69/1 -> Equal101/2
  Equal101/1 -> [SwPasReclinerEntryInt]
  SwPasReclinerEntryIntCnt/1 -> Unit Delay69/1, Equal101/1
  Equal102/1 -> [SwPasReclinerExitInt]
  Unit Delay70/1 -> Equal102/2
  SwPasReclinerExitIntCnt/1 -> Unit Delay70/1, Equal102/1
  SwUnfold3LIntCnt/1 -> Unit Delay71/1, Equal103/1
  Unit Delay71/1 -> Equal103/2
  Equal103/1 -> [SwUnfold3LInt]
  Equal104/1 -> [SwUnfold3RInt]
  Unit Delay72/1 -> Equal104/2
  SwUnfold3RIntCnt/1 -> Unit Delay72/1, Equal104/1
  Ground/1 -> SwIntAcsExt/1
  OR26/1 -> SwIntAcsEnty/1
  [Is2LStSwAct] -> OR26/1
  [Is2RStSwAct] -> OR26/2
  [Is3LStSwAct] -> OR26/3
  [Is3RStSwAct] -> OR26/4
  [SwAcsEntyLInt] -> OR26/5
  [SwAcsEntyRInt] -> OR26/6
  [SwAcsEntyBInt] -> OR26/7
  [SwLfVipInt] -> OR26/8
  [SwRtVipInt] -> OR26/9
  [SwLtLugInt] -> OR26/10
  [SwLtRcvyInt] -> OR26/11
  [SwRtRcvyInt] -> OR26/12
  [Is2LStSwAct] -> OR27/1
  [Is3LStSwAct] -> OR27/2
  [SwAcsEntyLInt] -> OR27/3
  [SwAcsEntyRInt] -> OR27/4
  [SwAcsEntyBInt] -> OR27/5
  [SwLfVipInt] -> OR27/6
  OR27/1 -> SwIntLfVip/1
  Switch3/1 -> OR28/4
  [Is3LStSwAct] -> Switch3/1
  Equal105/1 -> Switch3/2
  Constant37/1 -> Switch3/3
  Constant36/1 -> Equal105/2
  [SeStNumConfig] -> Equal105/1
  OR28/1 -> SwIntRtVip/1
  [IsPasStSwAct] -> OR28/1
  [Is2RStSwAct] -> OR28/2
  [Is3RStSwAct] -> OR28/3
  [SwAcsEntyLInt] -> OR28/5
  [SwAcsEntyRInt] -> OR28/6
  [SwAcsEntyBInt] -> OR28/7
  Ground1/1 -> SwIntLtFamily/1
  Ground2/1 -> SwIntIntimacyLt/1
  Ground3/1 -> SwIntIntimacyRt/1
  Constant39/1 -> Switch4/3
  Equal106/1 -> Switch4/2
  [SeStNumConfig] -> Equal106/1
  Constant38/1 -> Equal106/2
  [Is2LStSwAct] -> OR29/1
  [Is2RStSwAct] -> OR29/2
  OR29/1 -> Switch4/1
  Constant41/1 -> Switch5/3
  Equal107/1 -> Switch5/2
  [SeStNumConfig] -> Equal107/1
  Constant40/1 -> Equal107/2
  [SwRtVipInt] -> OR30/3
  OR30/1 -> Switch5/1
  [SwLtRcvyInt] -> OR30/1
  [SwRtRcvyInt] -> OR30/2
  Switch4/1 -> OR31/1
  [Is3LStSwAct] -> OR31/2
  [SwAcsEntyLInt] -> OR31/3
  [SwUnfold3LInt] -> OR31/9
  Switch5/1 -> OR31/7
  [SwLtLugInt] -> OR31/8
  [SwLfVipInt] -> OR31/6
  [SwAcsEntyBInt] -> OR31/5
  [SwAcsEntyRInt] -> OR31/4
  OR31/1 -> SwIntLfLug/1
  Constant42/1 -> Equal108/2
  [SeStNumConfig] -> Equal108/1
  Equal108/1 -> Switch6/2
  Constant43/1 -> Switch6/3
  [Is2RStSwAct] -> Switch6/1
  Equal109/1 -> Switch7/2
  [SeStNumConfig] -> Equal109/1
  Constant44/1 -> Equal109/2
  Constant45/1 -> Switch7/3
  [Is3RStSwAct] -> OR33/1
  Switch6/1 -> OR33/2
  [SwAcsEntyLInt] -> OR33/3
  [SwAcsEntyRInt] -> OR33/4
  [SwAcsEntyBInt] -> OR33/5
  [SwRtVipInt] -> OR33/6
  Switch7/1 -> OR33/7
  [SwRtLugInt] -> OR33/8
  OR33/1 -> SwIntRtLug/1
  Ground4/1 -> SwIntAcsEntryAll4sBwd/1, SwIntAcsEntryAll4sFwd/1
  Ground5/1 -> SwIntAcsExit4s2R/1
  Ground6/1 -> SwIntAcsEntry4s2R/1
  Ground7/1 -> SwIntAcsExit4s2L/1
  Ground8/1 -> SwIntAcsEntry4s2L/1
  Ground9/1 -> SwIntLgrstOpenRt/1
  Ground10/1 -> SwIntLgrstCloseRt/1
  Ground11/1 -> SwIntLgrstOpenLt/1
  Ground12/1 -> SwIntLgrstCloseLt/1
  Ground13/1 -> SwIntLtLying/1
  Ground14/1 -> SwIntRtLying/1
  Ground15/1 -> SwIntRtFamily/1
  [SwLtLugInt] -> Switch8/1
  Constant47/1 -> Switch8/3
  Equal110/1 -> Switch8/2
  [SeStNumConfig] -> Equal110/1
  Constant46/1 -> Equal110/2
  [Is2LStSwAct] -> OR34/1
  [SwAcsEntyLInt] -> OR34/2
  [SwUnfold3LInt] -> OR34/8
  Switch8/1 -> OR34/9
  [passCmprtMdHMIStop] -> OR34/7
  [SwLtRcvyInt] -> OR34/6
  [SwLfVipInt] -> OR34/5
  [SwAcsEntyBInt] -> OR34/4
  [SwAcsEntyRInt] -> OR34/3
  OR34/1 -> SwIntLfRcvy/1
  Constant48/1 -> Equal111/2
  [SeStNumConfig] -> Equal111/1
  Equal111/1 -> Switch9/2
  Constant49/1 -> Switch9/3
  [SwLtLugInt] -> Switch9/1
  [passCmprtMdHMIStop] -> OR35/10
  [SwUnfold3RInt] -> OR35/9
  [SwUnfold3LInt] -> OR35/8
  Switch9/1 -> OR35/7
  [SwRtRcvyInt] -> OR35/6
  [SwRtVipInt] -> OR35/5
  [SwAcsEntyBInt] -> OR35/4
  [SwAcsEntyRInt] -> OR35/3
  [SwAcsEntyLInt] -> OR35/2
  [Is2RStSwAct] -> OR35/1
  OR35/1 -> SwIntRtRcvy/1
  [SwUnfold3LInt] -> OR36/5
  [SwLtLugInt] -> OR36/4
  [SwAcsEntyBInt] -> OR36/3
  [SwAcsEntyRInt] -> OR36/2
  [SwAcsEntyLInt] -> OR36/1
  OR36/1 -> SwIntAllVip/1
  Constant57/1 -> Switch13/3
  Equal115/1 -> Switch13/2
  [SeStNumConfig] -> Equal115/1
  Constant56/1 -> Equal115/2
  OR38/1 -> Switch13/1
  Switch13/1 -> OR37/5
  [SwAllLugInt] -> OR37/4
  [SwAcsEntyBInt] -> OR37/3
  [SwAcsEntyRInt] -> OR37/2
  [SwAcsEntyLInt] -> OR37/1
  OR37/1 -> SwIntAllLug/1
  OR39/1 -> SwIntPasReclinerExit/1, SwIntPasReclinerEntry/1
  [IsPasStSwAct] -> OR39/1
  [Is2LStSwAct] -> OR40/1
  [Is2RStSwAct] -> OR40/2
  [Is3LStSwAct] -> OR40/3
  [SwAcsEntyLInt] -> OR40/4
  [SwRtRcvyInt] -> OR40/10
  [SwLtRcvyInt] -> OR40/9
  [SwRtVipInt] -> OR40/8
  [SwLfVipInt] -> OR40/7
  [SwAcsEntyBInt] -> OR40/6
  [SwAcsEntyRInt] -> OR40/5
  OR40/1 -> SwIntUnfold3L/1
  OR41/1 -> SwIntUnfold3R/1
  [Is2RStSwAct] -> OR41/1
  [Is3RStSwAct] -> OR41/2
  [SwAcsEntyLInt] -> OR41/3
  [SwAcsEntyRInt] -> OR41/4
  [SwAcsEntyBInt] -> OR41/5
  [SwRtVipInt] -> OR41/6
  [SwRtRcvyInt] -> OR41/7
  [SwLtLugInt] -> OR41/8
  [SwUnfold3LInt] -> OR26/13
  [SwUnfold3RInt] -> OR26/14
  [SwLtLugInt] -> OR40/11
  [SwUnfold3LInt] -> OR40/12
  AcsExtMdHMI2LRclReq/1 -> Terminator/1
  AcsExtMdHMI2RRclReq/1 -> Terminator1/1
  AcsEntryMdHMI2LRclReq/1 -> Terminator2/1
  AcsEntryMdHMI2RRclReq/1 -> Terminator3/1
  VipAllMdHMI2LRclReq/1 -> Terminator4/1
  VipAllMdHMI2RRclReq/1 -> Terminator5/1
  AllLugMdHMI2LRclReq/1 -> Terminator6/1
  AllLugMdHMI2RRclReq/1 -> Terminator7/1
  IntimacyLHMI2LRclReq/1 -> Terminator8/1
  IntimacyRHMI2RRclReq/1 -> Terminator9/1
  FamilyMdHMI2LRclReq/1 -> Terminator10/1
  FamilyMdHMI2RRclReq/1 -> Terminator11/1
  LtLugMdHMI2LRclReq/1 -> Terminator12/1
  RtLugMdHMI2RRclReq/1 -> Terminator13/1
  LtLyingMdHMI2LRclReq/1 -> Terminator14/1
  RtLyingMdHMI2RRclReq/1 -> Terminator15/1
  VIPMdHMI2LRclReq/1 -> Terminator16/1
  VIPMdHMI2RRclReq/1 -> Terminator17/1
  RcvyMdHMI2LRclReq/1 -> Terminator18/1
  RcvyMdHMI2RRclReq/1 -> Terminator19/1
  LgrstOpenLtHMI2LRclReq/1 -> Terminator20/1
  LgrstCloseLtHMI2LRclReq/1 -> Terminator21/1
  LgrstOpenRtHMI2RRclReq/1 -> Terminator22/1
  LgrstCloseRtHMI2RRclReq/1 -> Terminator23/1
  AcsEntry4s2LHMI2LRclReq/1 -> Terminator24/1
  AcsExit4s2LHMI2LRclReq/1 -> Terminator25/1
  AcsEntry4s2RHMI2RRclReq/1 -> Terminator26/1
  AcsExit4s2RHMI2RRclReq/1 -> Terminator27/1
  [passCmprtMdHMIStop] -> OR26/15
  [passCmprtMdHMIStop] -> OR36/6
  OR42/1 -> SwIntLfVipOut/1
  [SwLfVipInt] -> OR42/6
  [SwAcsEntyBInt] -> OR42/5
  [SwAcsEntyRInt] -> OR42/4
  [SwAcsEntyLInt] -> OR42/3
  [Is3LStSwAct] -> OR42/2
  [Is2LStSwAct] -> OR42/1
  [SwAcsEntyBInt] -> OR43/7
  [SwAcsEntyRInt] -> OR43/6
  [SwAcsEntyLInt] -> OR43/5
  [Is3RStSwAct] -> OR43/3
  [Is2RStSwAct] -> OR43/2
  [IsPasStSwAct] -> OR43/1
  [SeStNumConfig] -> Equal116/1
  Constant58/1 -> Equal116/2
  Constant59/1 -> Switch15/3
  Equal116/1 -> Switch15/2
  [Is3LStSwAct] -> Switch15/1
  Switch15/1 -> OR43/4
  OR43/1 -> SwIntRtVipOut/1
  [passCmprtMdHMIStop] -> OR44/6
  [SwAcsEntyLInt] -> OR44/1
  [SwAcsEntyRInt] -> OR44/2
  [SwAcsEntyBInt] -> OR44/3
  [SwLtLugInt] -> OR44/4
  OR44/1 -> SwIntAllVipOut/1
  [SwLtLugInt] -> OR27/7
  [SwLtRcvyInt] -> OR27/8
  [SwUnfold3LInt] -> OR27/9
  [passCmprtMdHMIStop] -> OR27/10
  [SwRtRcvyInt] -> OR28/9
  [SwRtVipInt] -> OR28/8
  [SwLtLugInt] -> OR28/10
  [SwUnfold3LInt] -> OR28/11
  [SwUnfold3RInt] -> OR28/12
  [SwPasReclinerEntryInt] -> OR28/14
  [passCmprtMdHMIStop] -> OR28/15
  [SwPasReclinerExitInt] -> OR28/13
  [SwLtLugInt] -> OR42/7
  [SwLtRcvyInt] -> OR42/8
  [SwUnfold3LInt] -> OR42/9
  [passCmprtMdHMIStop] -> OR42/10
  [SwRtVipInt] -> OR43/8
  [SwRtRcvyInt] -> OR43/9
  [SwLtLugInt] -> OR43/10
  [SwUnfold3LInt] -> OR43/11
  [passCmprtMdHMIStop] -> OR43/15
  [SwPasReclinerExitInt] -> OR43/13
  [SwPasReclinerEntryInt] -> OR43/14
  [SwUnfold3RInt] -> OR43/12
  [SwUnfold3LInt] -> OR44/5
  [SwRtVipInt] -> OR38/1
  [SwRtRcvyInt] -> OR38/2
  [passCmprtMdHMIStop] -> OR37/8
  [SwUnfold3LInt] -> OR37/6
  [SwUnfold3RInt] -> OR37/7
  [SwUnfold3RInt] -> OR41/9
  [SwRtVipInt] -> OR32/9
  [SwAcsEntyRInt] -> OR32/6
  [SwUnfold3LInt] -> OR32/13
  [Is3LStSwAct] -> OR32/3
  [SwUnfold3RInt] -> OR32/14
  [SwAcsEntyLInt] -> OR32/5
  [SwRtRcvyInt] -> OR32/12
  [SwLtRcvyInt] -> OR32/11
  [SwLfVipInt] -> OR32/8
  [SwLtLugInt] -> OR32/10
  [SwAcsEntyBInt] -> OR32/7
  [Is2LStSwAct] -> OR32/1
  [Is2RStSwAct] -> OR32/2
  [Is3RStSwAct] -> OR32/4
  OR32/1 -> SwIntBig4Seat/1
  [passCmprtMdHMIStop] -> OR31/10
  [passCmprtMdHMIStop] -> OR33/11
  [SwUnfold3RInt] -> OR33/10
  [SwUnfold3LInt] -> OR33/9
  [SwUnfold3RInt] -> OR31/11
  [passCmprtMdHMIStop] -> OR45/15
  [SwRtVipInt] -> OR45/8
  [SwPasReclinerEntryInt] -> OR45/14
  [SwLtLugInt] -> OR45/10
  [SwUnfold3RInt] -> OR45/12
  [SwPasReclinerExitInt] -> OR45/13
  [SwUnfold3LInt] -> OR45/11
  [Is3RStSwAct] -> OR45/3
  [SeStNumConfig] -> Equal112/1
  [SwAcsEntyRInt] -> OR45/6
  [SwAcsEntyBInt] -> OR45/7
  [SwAcsEntyLInt] -> OR45/5
  [Is2RStSwAct] -> OR45/2
  [SwRtRcvyInt] -> OR45/9
  Constant50/1 -> Equal112/2
  Equal112/1 -> Switch10/2
  [IsPasStSwAct] -> OR45/1
  Switch10/1 -> OR45/4
  [Is3LStSwAct] -> Switch10/1
  Constant51/1 -> Switch10/3
  OR45/1 -> SwIntExVIPR/1
  [SwAcsEntyBInt] -> OR46/7
  [SwAcsEntyRInt] -> OR46/6
  [SwLtLugInt] -> OR46/10
  [SeStNumConfig] -> Equal113/1
  [SwRtVipInt] -> OR46/8
  [SwUnfold3LInt] -> OR46/11
  [Is3RStSwAct] -> OR46/3
  Constant52/1 -> Equal113/2
  [SwUnfold3RInt] -> OR46/12
  [SwPasReclinerEntryInt] -> OR46/14
  [SwAcsEntyLInt] -> OR46/5
  Switch11/1 -> OR46/4
  [passCmprtMdHMIStop] -> OR46/15
  [IsPasStSwAct] -> OR46/1
  Equal113/1 -> Switch11/2
  Constant53/1 -> Switch11/3
  [SwPasReclinerExitInt] -> OR46/13
  [Is2RStSwAct] -> OR46/2
  [SwRtRcvyInt] -> OR46/9
  [Is3LStSwAct] -> Switch11/1
  OR46/1 -> SwIntExVIPROut/1
  [SwPasReclinerEntryInt] -> OR39/5
  [SwPasReclinerExitInt] -> OR39/4
  [SwRtVipInt] -> OR39/3
  [Is2RStSwAct] -> OR39/2
  [SwPasReclinerExitInt] -> OR26/16
  [SwPasReclinerEntryInt] -> OR26/17
  [SwPasReclinerExitInt] -> OR30/4
  [SwPasReclinerEntryInt] -> OR30/5
  [SwPasReclinerExitInt] -> OR47/1
  [SwPasReclinerEntryInt] -> OR47/2
  [SwRtRcvyInt] -> OR47/3
  OR47/1 -> Switch7/1
  [SwPasReclinerExitInt] -> OR35/11
  [SwPasReclinerEntryInt] -> OR35/12
  [SwPasReclinerExitInt] -> OR40/13
  [SwPasReclinerEntryInt] -> OR40/14
  [passCmprtMdHMIStop] -> OR40/15
  [passCmprtMdHMIStop] -> OR41/12
  [SwPasReclinerExitInt] -> OR41/10
  [SwPasReclinerEntryInt] -> OR41/11
  [passCmprtMdHMIStop] -> OR32/17
  [SwPasReclinerExitInt] -> OR32/16
  [SwPasReclinerEntryInt] -> OR32/15
  OR48/1 -> Switch12/1
  Constant55/1 -> Switch12/3
  Constant54/1 -> Equal114/2
  [SeStNumConfig] -> Equal114/1
  Equal114/1 -> Switch12/2
  [SwUnfold3LInt] -> OR39/6
  [SwUnfold3RInt] -> OR39/7
  [SwAllLugInt] -> OR48/1
  [SwRtLugInt] -> OR48/2
  [SwLtLugInt] -> OR48/3
  [SwRtRcvyInt] -> OR39/8
  [SwAcsEntyLInt] -> OR39/9
  [SwAcsEntyRInt] -> OR39/10
  [SwAcsEntyBInt] -> OR39/11
  Switch12/1 -> OR39/12
  [passCmprtMdHMIStop] -> OR39/13
  OR49/1 -> SwIntWholeVehMem2/1, SwIntWholeVehMem1/1
  [IsPasStSwAct] -> OR49/1
  [Is2LStSwAct] -> OR49/2
  [Is2RStSwAct] -> OR49/3
  [Is3LStSwAct] -> OR49/4
  [Is3RStSwAct] -> OR49/5
  [SwAcsEntyLInt] -> OR49/6
  [SwUnfold3RInt] -> OR49/19
  [passCmprtMdHMIStop] -> OR49/20
  [SwUnfold3LInt] -> OR49/18
  [SwPasReclinerExitInt] -> OR49/17
  [SwPasReclinerEntryInt] -> OR49/16
  [SwRtRcvyInt] -> OR49/15
  [SwLtRcvyInt] -> OR49/14
  [SwLtLugInt] -> OR49/13
  [SwRtLugInt] -> OR49/12
  [SwAllLugInt] -> OR49/11
  [SwRtVipInt] -> OR49/10
  [SwLfVipInt] -> OR49/9
  [SwAcsEntyBInt] -> OR49/8
  [SwAcsEntyRInt] -> OR49/7
  [SwPasReclinerExitInt] -> OR38/3
  [SwPasReclinerEntryInt] -> OR38/4
